simulink model "LQG_longitudinal"  (R2016b)
settings: Solver=VariableStepAuto  StartTime=0.0  StopTime=20  RelTol=1e-3
undefined symbols (not defined in the file or in its folder): A_long, B_long, C_long, Continuous, D_long, K_long, Time
libraries: dspsrcs4 x1, ctrlSharedLib x1
settings Model: Creator=yashm  LastModifiedBy=yashm

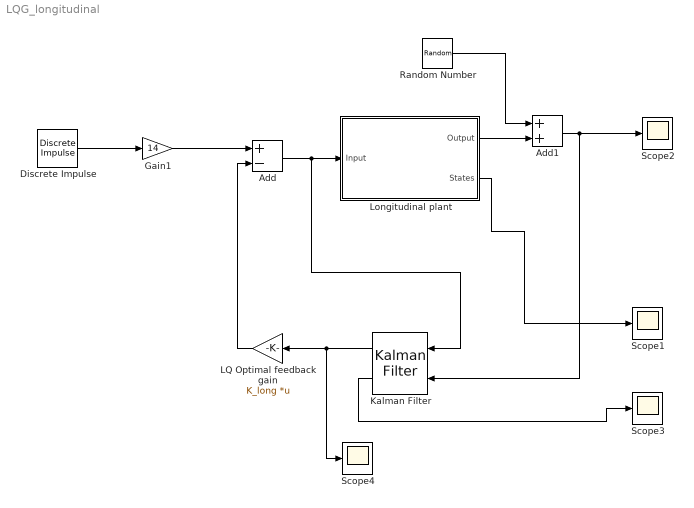
== system LQG_longitudinal ==
  Add : Sum  Inputs=+-
  Add1 : Sum
  Discrete Impulse : dspsrcs4/Discrete  Impulse  Delay=0  SampleTime=1  FrameSample=1  OutputFrames=off  dataType=double  isSigned=on  wordLen=16  udDataType=sfix(16)  fracBitsMode=Best precision  numFracBits=15  OutDataTypeStr=double  LastOutDataTypeStr=double
  Gain1 : Gain  Gain=14
  Kalman Filter : ctrlSharedLib/Kalman Filter  TimeDomain=Continuous-Time  UseCurrentEstimator=on  ModelSource=Individual A, B, C, D matrices  ModelSourceVariable=ss(0.95,1,1,0,1)  A=A_long  B=B_long  C=C_long  D=D_long  NumberOfStates=1  NumberOfInputs=1  NumberOfOutputs=1  InitialEstimateSource=Dialog  X0=0  P0=10  UseK=off  UseGH=off  NumberOfProcessNoiseInputs=1  G=1  TimeInvariantG=on  H=0  TimeInvariantH=on  Q=1  TimeInvariantQ=on  R=1  TimeInvariantR=on  N=0  TimeInvariantN=on  AddInputPort=on  AddEnablePort=off  ExternalReset=none  OutputEstimatedY=on  OutputP=off  Ts=0.01
  LQ Optimal feedback gain : Gain  Gain=K_long  Multiplication=Matrix(K*u)
  Longitudinal plant : Subsystem
  Random Number : RandomNumber  Variance=1e-5  SampleTime=0.01
  Scope{1..4} (4 alike) : Scope
  wires:
  Add/1 -> Kalman Filter/1, Longitudinal plant/1(Input)
  Longitudinal plant/2(States) -> Scope1/1
  LQ Optimal feedback gain/1 -> Add/2
  Gain1/1 -> Add/1
  Discrete Impulse/1 -> Gain1/1
  Kalman Filter/1 -> Scope4/1, LQ Optimal feedback gain/1
  Longitudinal plant/1(Output) -> Add1/2
  Random Number/1 -> Add1/1
  Add1/1 -> Kalman Filter/2, Scope2/1
  Kalman Filter/2 -> Scope3/1

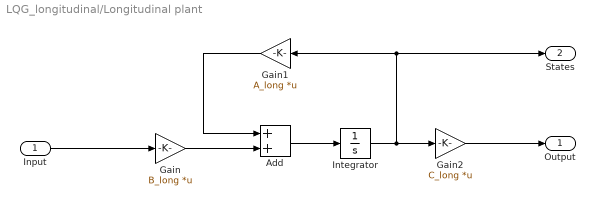
== system LQG_longitudinal/Longitudinal plant ==
  Input : Inport
  Add : Sum
  Gain : Gain  Gain=B_long  Multiplication=Matrix(K*u)
  Gain1 : Gain  Gain=A_long  Multiplication=Matrix(K*u)
  Gain2 : Gain  Gain=C_long  Multiplication=Matrix(K*u)
  Integrator : Integrator
  Output : Outport
  States : Outport  Port=2
  wires:
  Gain2/1 -> Output/1
  Input/1 -> Gain/1
  Gain/1 -> Add/2
  Integrator/1 -> Gain1/1, States/1, Gain2/1
  Add/1 -> Integrator/1
  Gain1/1 -> Add/1
